simulink model "trim_helper"  (R2016a)
settings: Solver=VariableStepAuto  StartTime=0.0  StopTime=10.0  RelTol=1e-3
values from neighbouring files (symbols this model uses):
  x0 = [0 0  x0(3)         phi0     theta0    psi0   Va  0  0   0   0   0  ]'    [simX8.m]
settings Model: Creator=krisgry  LastModifiedBy=krisgry

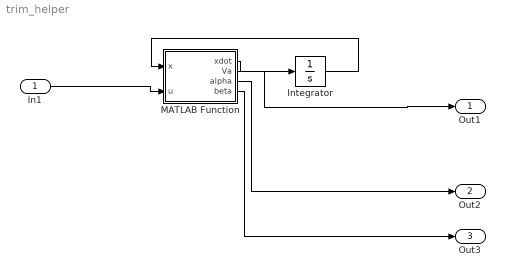
== system trim_helper ==
  In1 : Inport
  Integrator : Integrator  InitialCondition=x0
  MATLAB Function : MATLAB Function  TreatAsAtomicUnit=on
  Out1 : Outport
  Out2 : Outport  Port=2
  Out3 : Outport  Port=3
  wires:
  MATLAB Function/1(xdot) -> Integrator/1
  Integrator/1 -> MATLAB Function/1(x)
  In1/1 -> MATLAB Function/2(u)
  MATLAB Function/2(Va) -> Out1/1
  MATLAB Function/3(alpha) -> Out2/1
  MATLAB Function/4(beta) -> Out3/1

== matlab function trim_helper/MATLAB Function ==
  data: x input size=12; u input size=4; xdot output size=12; P parameter; Va output; alpha output; beta output
function [xdot,Va,alpha,beta] = fcn(x,u,P)
%#codegen

xdot = dynamics(0,x,P,forces(0,x,P,u,zeros(6,1)));

Va = norm(x(7:9)); %airspeed
alpha = atan(x(9)/x(7)); %no wind
beta = asin(x(8)/Va); %no wind
